simulink model "Microgrid_w_BESS"  (R2024b)
settings: Solver=VariableStepAuto  StartTime=0.0  StopTime=4  RelTol=1e-3
undefined symbols (not defined in the file or in its folder): Ion, Lithium, Ts_Control
libraries: spsParallelRLCBranchLib x8, simulink x6, spsSeriesRLCBranchLib x6, powerlib_extras x6, ee_lib x5, nesl_utility x5, slpidlib x5, spsThreePhaseVIMeasurementLib x3, spsThreePhaseSeriesRLCBranchLib x3, spsCurrentVoltageSimscapeInterfaceLib x3, eePowerMeasurement x3, spsVoltageMeasurementLib x2
(part 1 of 2)
settings Model: Creator=DELL  LastModifiedBy=mitphanase
settings DataIOCC: ReturnWorkspaceOutputs=off

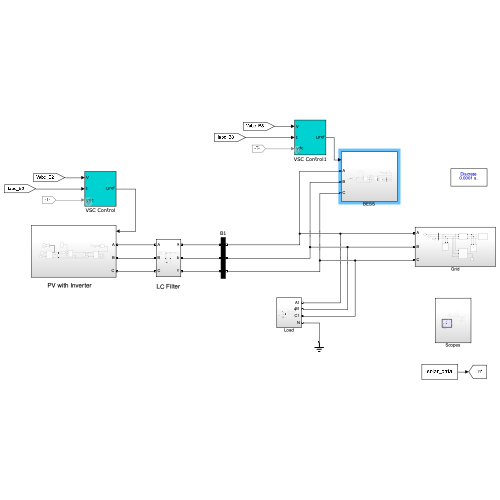
[thumbnail: Simulink's stored preview of the top-level diagram]
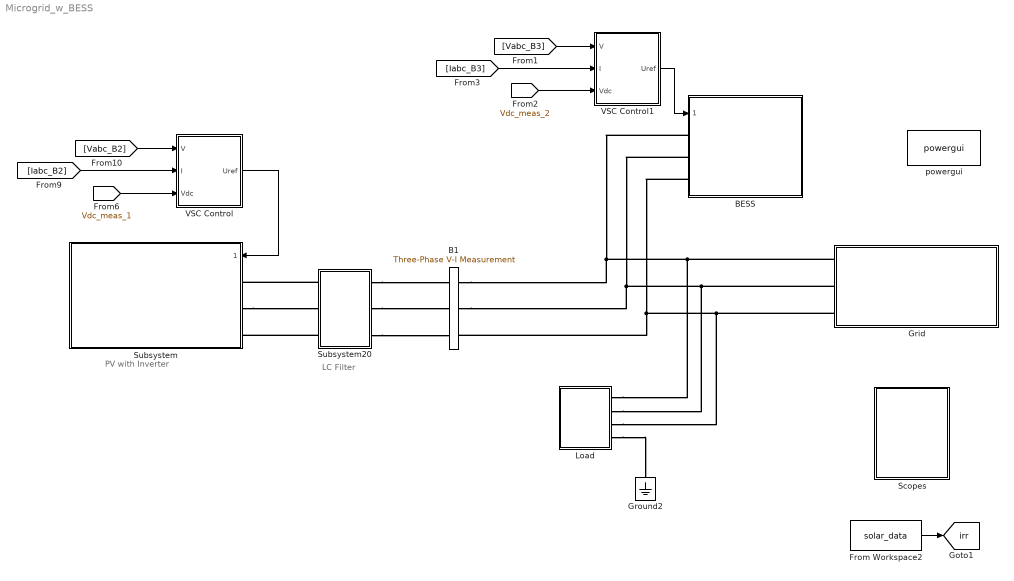
== system Microgrid_w_BESS ==
  note: LC Filter
  note: PV with Inverter
  B1 : spsThreePhaseVIMeasurementLib/Three-Phase V-I Measurement  VoltageMeasurement=phase-to-ground  SetLabelV=on  LabelV=Vabc_B1  Vpu=off  VpuLL=off  CurrentMeasurement=yes  SetLabelI=on  LabelI=Iabc_B1  Ipu=off  Pbase=100e6  Vbase=1000  OutputType=Magnitude  PhasorSimulation=off  PSBequivalent=0
  BESS : Subsystem
  From Workspace2 : FromWorkspace  VariableName=solar_data  OutDataTypeStr=double  SampleTime=0.01
  Grid : Subsystem
  Ground2 : spsGroundLib/Ground  LConnTagsString=a
  Load : Subsystem
  Scopes : Subsystem
  Subsystem : Subsystem
  Subsystem20 : Subsystem
  VSC Control : Subsystem  mask(VSC Main Controller){nom=[ 50e3  50 ], Vnom=[ 400 400 ], Vnom_dc=700, RLxfo=[0  0 ], RLchoke=[0  0  ], K_VDCreg=[18  600], K_Ireg=[0.2 20], Ts=Ts_Control}
      mask prompts: nom "Nominal power and frequency [ Pnom(VA)  Fnom(Hz) ]:"; Vnom "Nominal primary and secondary voltages (Vrms LL) [ Vnom_prim   Vnom_sec ]:"; Vnom_dc "Nominal DC bus voltage (V):"; RLxfo "Total transformer leakage impedance (pu/Pnom) [ Rxfo  Lxf ]"; RLchoke "Choke impedance [ R(ohm) L(H) ]"; K_VDCreg "VDC regultator gains [ Kp  Ki ]:"; K_Ireg "Current regulator gains [ Kp  Ki ]:"; Ts "Sample time"
      mask init:
      | Pnom=nom(1);
      | Fnom=nom(2);
      | Vnom_prim=Vnom(1);
      | Vnom_sec=Vnom(2);
      | Zbase=Vnom_sec^2/Pnom;
      | Rtot_pu=RLxfo(1) + RLchoke(1)/Zbase;
      | Ltot_pu=RLxfo(2) + RLchoke(2)/(Zbase/(2*pi*Fnom));
      | Kp_VDCreg=K_VDCreg(1);
      | Ki_VDCreg=K_VDCreg(2);
      | Kp_Ireg=K_Ireg(1);
      | Ki_Ireg=K_Ireg(2);
      | Vdc_ref=Vnom_dc;
  VSC Control1 : Subsystem  mask(VSC Main Controller){nom=[ 45e3  50 ], Vnom=[ 400 400 ], Vnom_dc=600, RLxfo=[0  0 ], RLchoke=[0  0  ], K_VDCreg=[18  600], K_Ireg=[0.2 20], Ts=Ts_Control}
      mask prompts: nom "Nominal power and frequency [ Pnom(VA)  Fnom(Hz) ]:"; Vnom "Nominal primary and secondary voltages (Vrms LL) [ Vnom_prim   Vnom_sec ]:"; Vnom_dc "Nominal DC bus voltage (V):"; RLxfo "Total transformer leakage impedance (pu/Pnom) [ Rxfo  Lxf ]"; RLchoke "Choke impedance [ R(ohm) L(H) ]"; K_VDCreg "VDC regultator gains [ Kp  Ki ]:"; K_Ireg "Current regulator gains [ Kp  Ki ]:"; Ts "Sample time"
      mask init: same as Microgrid_w_BESS/VSC Control
  powergui : sps_lib/powergui  Priority=1  SimulationMode=Discrete  SampleTime=1e-4  frequency=60  Iterations=50  frequencyindice=0  Pbase=100e6  ErrMax=1e-4  UnitsV=kV  UnitsW=MW  buscounter=0  FunctionMessages=off  echomessages=off  EnableUseOfTLC=off  CurrentSourceSwitches=off  DisableSnubberDevices=off  DisableRonSwitches=off  DisableVfSwitches=off  DisplayEquations=off  AutomaticDiscreteSolvers=off  SolverType=Tustin/Backward Euler (TBE)  Interpol=off  ExternalGateDelay=off  methode=off  Ts=100  x0status=blocks  SPID=on  SwTol=0  HookPort=off  NonlinearTolerance=1e-4  nMaxIteration=100  ContinueOnMaxIteration=off  RestoreLinks=warning  ResistiveCurrentMeasurement=off  Frange=[0:2:500]  Ylog=off  Xlog=on  ShowGrid=off  save=off  variable=ZData  structure=0  ZoomFFT=off  StartTime=0.0  cycles=1  DisplayStyle=1  fundamental=60  FreqAxis=off  MaxFrequency=1000  frequencyindicesteady=1  RmsSteady=1  display=off
  tag scope: irr=global
  wires:
  [Vdc_meas_1] -> VSC Control/3(Vdc)
  [Vabc_B2] -> VSC Control/1(V)
  [Iabc_B2] -> VSC Control/2(I)
  VSC Control/1(Uref) -> Subsystem/1("  ")
  From Workspace2/1 -> [irr]
  [Iabc_B3] -> VSC Control1/2(I)
  [Vabc_B3] -> VSC Control1/1(V)
  [Vdc_meas_2] -> VSC Control1/3(Vdc)
  VSC Control1/1(Uref) -> BESS/1("  ")
  connections:
  Grid/LConn1 -- Load/LConn1 -- B1/RConn1 -- BESS/LConn1
  Grid/LConn3 -- Load/LConn3 -- BESS/LConn3 -- B1/RConn3
  Grid/LConn2 -- Load/LConn2 -- B1/RConn2 -- BESS/LConn2
  Subsystem20/LConn1 -- Subsystem/LConn1
  Subsystem/LConn2 -- Subsystem20/LConn2
  Subsystem20/LConn3 -- Subsystem/LConn3
  Subsystem20/RConn1 -- B1/LConn1
  Subsystem20/RConn2 -- B1/LConn2
  Subsystem20/RConn3 -- B1/LConn3
  Load/LConn4 -- Ground2/LConn1

== system Microgrid_w_BESS/BESS ==
  "  " : Inport
  B3 : spsThreePhaseVIMeasurementLib/Three-Phase V-I Measurement  VoltageMeasurement=phase-to-ground  SetLabelV=on  LabelV=Vabc_B3  Vpu=off  VpuLL=off  CurrentMeasurement=yes  SetLabelI=on  LabelI=Iabc_B3  Ipu=off  Pbase=100e6  Vbase=1000  OutputType=Magnitude  PhasorSimulation=off  PSBequivalent=0
  BATT chg-dshg logic1 : Subsystem
  Battery : spsBatteryLib/Battery  BatType=Lithium-Ion  NomV=400  NomQ=150  SOC=0  Batt_Tr=0.01  PresetModel=on  MaxQ=150  MinV=300  FullV=465.5949  Dis_rate=65.2174  R=0.026667  Normal_OP=135.6522  expZone="[432.1543      7.369565]"
  Current Measurement : spsCurrentMeasurementLib/Current Measurement  PhasorSimulation=off  OutputType=Complex  PSBequivalent=0
  Inverter ON/OFF Logic : Subsystem
  L_B : spsSeriesRLCBranchLib/Series RLC Branch  LConnTagsString=__new0  RConnTagsString=__new0  BranchType=L  Resistance=5e-3  Inductance=1e-3  SetiL0=off  InitialCurrent=0  Capacitance=100e-6  Setx0=off  InitialVoltage=230  Measurements=None
  Subsystem : Subsystem
  Subsystem20 : Subsystem
  Two-Level Converter : spsTwoLevelConverterLib/Two-Level Converter  ModelType=Average model (No rectifier mode)  Ron=1e-3  Rs=1e6  Cs=inf  Vforward=[0,0]  Ron_Diode=1e-3  Rs_Diode=1e6  Cs_Diode=inf  Vf_Diode=1e-3  Rs_CurrentSource=inf  Ron_ACsource=1e-3
      settings: LibrarySourceBlock=sps_lib/Power Electronics/Two-Level Converter
  Two-Quadrant DC/DC Converter : spsTwoQuadrantDCDCConverterLib/Two-Quadrant DC//DC Converter  ModelType=Average model (D-controlled)  Ron=1e-3  Rs=1e6  Cs=inf  Vforward=[0,0]  Ron_Diode=1e-3  Rs_Diode=1e6  Cs_Diode=inf  Vf_Diode=1e-3  Rs_CurrentSource=inf  Ron_ACsource=1e-3
  A : PMIOPort  Side=Left
  B : PMIOPort  Port=2  Side=Left
  C : PMIOPort  Port=3  Side=Left
  tag scope: Batt_m=global
  wires:
  BATT chg-dshg logic1/1(D) -> Two-Quadrant DC/DC Converter/1
  [Vdc_meas_2] -> Inverter ON/OFF Logic/1(V_DC)
  "  "/1 -> Inverter ON/OFF Logic/2(g_in)
  Inverter ON/OFF Logic/1(g_out) -> Two-Level Converter/1
  Battery/1 -> [Batt_m]
  connections:
  Two-Level Converter/RConn2 -- Subsystem/RConn2 -- Two-Quadrant DC/DC Converter/RConn2 -- Battery/LConn2
  L_B/RConn1 -- Two-Quadrant DC/DC Converter/LConn1
  Subsystem/RConn1 -- Two-Level Converter/RConn1 -- Two-Quadrant DC/DC Converter/RConn1
  Subsystem20/LConn2 -- Two-Level Converter/LConn2
  Two-Level Converter/LConn1 -- Subsystem20/LConn1
  Two-Level Converter/LConn3 -- Subsystem20/LConn3
  Current Measurement/RConn1 -- Battery/LConn1
  Current Measurement/LConn1 -- L_B/LConn1
  B3/LConn1 -- Subsystem20/RConn1
  B3/LConn2 -- Subsystem20/RConn2
  B3/LConn3 -- Subsystem20/RConn3
  B3/RConn1 -- A/RConn1
  B3/RConn2 -- B/RConn1
  B3/RConn3 -- C/RConn1

== system Microgrid_w_BESS/Grid ==
  B2 : spsThreePhaseVIMeasurementLib/Three-Phase V-I Measurement  VoltageMeasurement=phase-to-ground  SetLabelV=on  LabelV=Vabc_B2  Vpu=off  VpuLL=off  CurrentMeasurement=yes  SetLabelI=on  LabelI=Iabc_B2  Ipu=off  Pbase=100e6  Vbase=500e3  OutputType=Magnitude  PhasorSimulation=off  PSBequivalent=0
  Ground : spsGroundLib/Ground  LConnTagsString=a
  "Grounding Transformer " : spsGroundingTransformerLib/Grounding Transformer   UNITS=SI  NominalPower="[3e3   50]"  NominalVoltage=0.4e3  ZeroSequenceImpedance_pu=[0.025 0.75]  MagnetizationBranch_pu=[500 500]  ZeroSequenceImpedance_SI=[1.3333 40]  MagnetizationBranch_SI=[26667 26667]  Measurements=All voltages and currents
      settings: LibrarySourceBlock=|
      | sps_lib/Power Grid Elements/Grounding
      | Transformer
  Three-Phase Series RLC Branch3 : spsThreePhaseSeriesRLCBranchLib/Three-Phase Series RLC Branch  LConnTagsString=A|B|C  RConnTagsString=A|B|C  BranchType=RL  Resistance=0.02  Inductance=1e-3  Capacitance=1e-6  Measurements=None
  Three-Phase Series RLC Load : spsThreePhaseSeriesRLCLoadLib/Three-Phase Series RLC Load  LConnTagsString=A|B|C  Configuration=Y (grounded)  NominalVoltage=400  Vabc=[1e3 1e3 1e3]  Vabcp=[1e3 1e3 1e3]  NominalFrequency=50  UnbalancedPower=off  ActivePower=0.1  InductivePower=0  CapacitivePower=100  Pabc=[10e3 9e3 11e3]  QLabc=[100 90 110]  QCabc=[100 90 110]  Pabcp=[10e3 9e3 11e3]  QLabcp=[100 90 110]  QCabcp=[100 90 110]  Measurements=None  LoadType=constant Z
  Three-Phase Series RLC Load1 : spsThreePhaseSeriesRLCLoadLib/Three-Phase Series RLC Load  LConnTagsString=A|B|C  Configuration=Y (grounded)  NominalVoltage=400  Vabc=[1e3 1e3 1e3]  Vabcp=[1e3 1e3 1e3]  NominalFrequency=50  UnbalancedPower=off  ActivePower=10  InductivePower=0  CapacitivePower=0  Pabc=[10e3 9e3 11e3]  QLabc=[100 90 110]  QCabc=[100 90 110]  Pabcp=[10e3 9e3 11e3]  QLabcp=[100 90 110]  QCabcp=[100 90 110]  Measurements=None  LoadType=constant Z
  Three-Phase Source : spsThreePhaseSourceLib/Three-Phase Source  InternalConnection=Yg  VoltagePhases=off  Voltage=400  PhaseAngle=0  Voltage_phases=[25e3 25e3 25e3]/sqrt(3)  PhaseAngles_phases=[0 -120 +120]  Frequency=50  NonIdealSource=on  SpecifyImpedance=on  Resistance=0.0113  Inductance=36e-6  ShortCircuitLevel=10e6  BaseVoltage=400  XRratio=6  BusType=swing  Pref=10e3  Qref=0  Prefabc=[10e3, 10e3, 10e3]  Qrefabc=[0, 0, 0]  Qmin=-inf  Qmax=inf
  A : PMIOPort  Side=Left
  B : PMIOPort  Port=2  Side=Left
  C : PMIOPort  Port=3  Side=Left
  connections:
  "Grounding Transformer "/RConn1 -- Ground/LConn1
  Three-Phase Series RLC Load/LConn1 -- Three-Phase Series RLC Branch3/RConn1 -- Three-Phase Source/RConn1
  Three-Phase Series RLC Load/LConn2 -- Three-Phase Series RLC Branch3/RConn2 -- Three-Phase Source/RConn2
  Three-Phase Series RLC Load/LConn3 -- Three-Phase Series RLC Branch3/RConn3 -- Three-Phase Source/RConn3
  "Grounding Transformer "/LConn1 -- B2/LConn1 -- Three-Phase Series RLC Load1/LConn1 -- Three-Phase Series RLC Branch3/LConn1
  "Grounding Transformer "/LConn2 -- Three-Phase Series RLC Load1/LConn2 -- B2/LConn2 -- Three-Phase Series RLC Branch3/LConn2
  "Grounding Transformer "/LConn3 -- Three-Phase Series RLC Load1/LConn3 -- B2/LConn3 -- Three-Phase Series RLC Branch3/LConn3
  B2/RConn3 -- C/RConn1
  B2/RConn2 -- B/RConn1
  B2/RConn1 -- A/RConn1

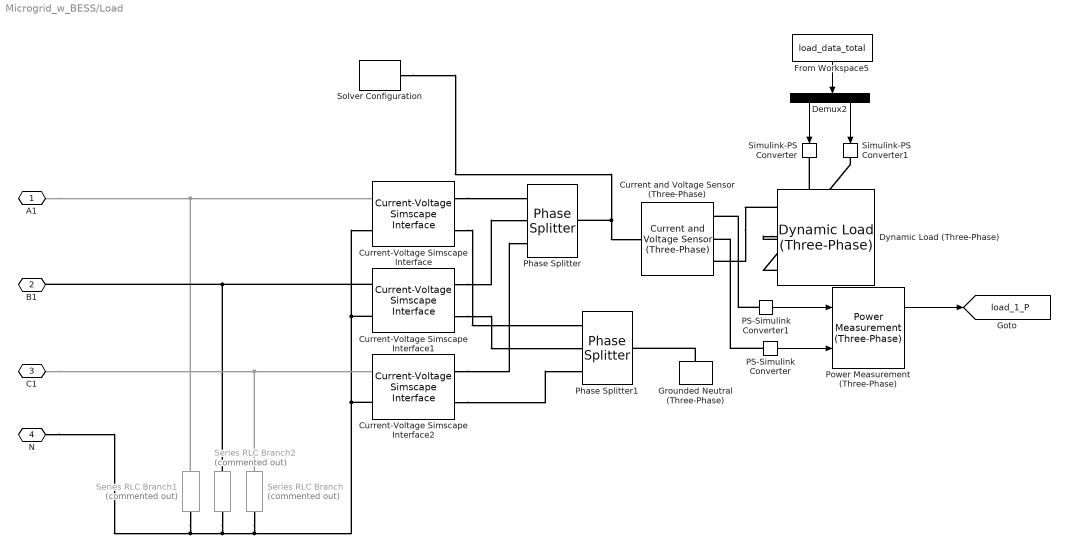
== system Microgrid_w_BESS/Load ==
  Current and Voltage Sensor (Three-Phase) : ee_lib/Sensors & Transducers/Current and Voltage Sensor (Three-Phase)  vMeasurementType=ee.enum.vmeasurement.ll  outputUnit=ee.enum.unit.si  SRated=100e6 A*V  VRated=24e3 V  I_specify=off  I_priority=None  I=[0, 0, 0] A  I_nominal_specify=off  I_nominal_value=1  I_nominal_unit=A  V_specify=off  V_priority=None  V=[0, 0, 0] V  V_nominal_specify=off  V_nominal_value=1  V_nominal_unit=V
      settings: InternalSimscapePortConfiguration="{\"Bottom\":[],\"Left\":[{\"id\":\"N1\",\"label\":\"~1\",\"type\":\"foundation.electrical.three_phase\"}],\"Right\":[{\"id\":\"V_output\",\"label\":\"V\",\"type\":\"output\"},{\"id\":\"I_output\",\"label\":\"I\",\"type\":\"output\"},{\"id\":\"N2\",\"label\":\"~2\",\"type\":\"foundation.electrical.three_phase\"}],\"Top\":[]}"
  Current-Voltage Simscape Interface : spsCurrentVoltageSimscapeInterfaceLib/Current-Voltage Simscape Interface  DFT=off  FMode=Low pass filter (continuous)  T=1e-4  Ts=50e-6  i0=0  v0=0  Sd=Specialized Power Systems side  Measurements=off
  Current-Voltage Simscape Interface1 : spsCurrentVoltageSimscapeInterfaceLib/Current-Voltage Simscape Interface  DFT=off  FMode=Low pass filter (continuous)  T=1e-4  Ts=50e-6  i0=0  v0=0  Sd=Specialized Power Systems side  Measurements=off
  Current-Voltage Simscape Interface2 : spsCurrentVoltageSimscapeInterfaceLib/Current-Voltage Simscape Interface  DFT=off  FMode=Low pass filter (continuous)  T=1e-4  Ts=50e-6  i0=0  v0=0  Sd=Specialized Power Systems side  Measurements=off
  Demux2 : Demux  Outputs=2
  Dynamic Load (Three-Phase) : ee_lib/Passive/Dynamic Load (Three-Phase)  port_option=ee.enum.threePhasePort.composite  FRated=50 Hz  Vline_rms_min=1 V  tau=0.01 s  Vline_rms_ini=400 V  Vang_ini=0 deg  gmin=0 S  fault_action=simscape.enum.assert.action.none  t_fault=1 s
      settings: InternalSimscapePortConfiguration="{\"Bottom\":[],\"Left\":[{\"id\":\"N\",\"label\":\"~\",\"type\":\"foundation.electrical.three_phase\"}],\"Right\":[],\"Top\":[{\"id\":\"P\",\"label\":\"P\",\"type\":\"input\"},{\"id\":\"Q\",\"label\":\"Q\",\"type\":\"input\"}]}"
  From Workspace5 : FromWorkspace  VariableName=load_data_total  SampleTime=0.01
  Grounded Neutral (Three-Phase) : ee_lib/Connectors & References/Grounded Neutral (Three-Phase)
  PS-Simulink Converter : nesl_utility/PS-Simulink Converter  PhysicalDomain=network_engine_domain  SubClassName=ps_output  LeftPortType=input  RightPortType=output  PseudoPeriodic=off  Frequencies=[]  VectorFormat=inherit  Unit=inherit  AffineConversion=off
  PS-Simulink Converter1 : nesl_utility/PS-Simulink Converter  PhysicalDomain=network_engine_domain  SubClassName=ps_output  LeftPortType=input  RightPortType=output  PseudoPeriodic=off  Frequencies=[]  VectorFormat=inherit  Unit=inherit  AffineConversion=off
  Phase Splitter : ee_lib/Connectors & References/Phase Splitter
  Phase Splitter1 : ee_lib/Connectors & References/Phase Splitter
  Power Measurement (Three-Phase) : eePowerMeasurement/Power Measurement (Three-Phase)  LabelModeActiveChoice=Discrete  F=50  K=[1]  Seq=Positive  Ts=0.01
  Series RLC Branch : spsSeriesRLCBranchLib/Series RLC Branch  Commented=on  LConnTagsString=__new0  RConnTagsString=__new0  BranchType=R  Resistance=1  Inductance=1e-3  SetiL0=off  InitialCurrent=0  Capacitance=1e-6  Setx0=off  InitialVoltage=0  Measurements=None
  Series RLC Branch1 : spsSeriesRLCBranchLib/Series RLC Branch  Commented=on  LConnTagsString=__new0  RConnTagsString=__new0  BranchType=R  Resistance=1  Inductance=1e-3  SetiL0=off  InitialCurrent=0  Capacitance=1e-6  Setx0=off  InitialVoltage=0  Measurements=None
  Series RLC Branch2 : spsSeriesRLCBranchLib/Series RLC Branch  Commented=on  LConnTagsString=__new0  RConnTagsString=__new0  BranchType=R  Resistance=1  Inductance=1e-3  SetiL0=off  InitialCurrent=0  Capacitance=1e-6  Setx0=off  InitialVoltage=0  Measurements=None
  Simulink-PS Converter : nesl_utility/Simulink-PS Converter  PhysicalDomain=network_engine_domain  SubClassName=ps_input  LeftPortType=input  RightPortType=output  PseudoPeriodic=off  Frequencies=[]  NoiseDistribution=none  NoiseParameters=[]  Unit=1  AffineConversion=off  FilteringAndDerivatives=provide  SimscapeFilterOrder=1  InputFilterTimeConstant=0.001  UdotUserProvided=0
  Simulink-PS Converter1 : nesl_utility/Simulink-PS Converter  PhysicalDomain=network_engine_domain  SubClassName=ps_input  LeftPortType=input  RightPortType=output  PseudoPeriodic=off  Frequencies=[]  NoiseDistribution=none  NoiseParameters=[]  Unit=1  AffineConversion=off  FilteringAndDerivatives=provide  SimscapeFilterOrder=1  InputFilterTimeConstant=0.001  UdotUserProvided=0
  Solver Configuration : nesl_utility/Solver Configuration  PhysicalDomain=network_engine_domain  SubClassName=solver  LeftPortType=input  RightPortType=generic  Tones=[]  Harmonics=[]  SimulateNoise=off  Profile=off  UseLocalSampling=off  EnableSwitchedLinearOptims=on  FrequencyDomain=off  UseCCode=off  RelTol=0.001  AbsTol=0.001  MinStep=1e-09  ToWorkspace=off  RevertToSquareIcSolve=off  NumHomotopyIterations=100  PhasorMode=off  PhasorModeNumHarmonics=1  ConsistencySolver=NEWTON_XTOL_AFTER_FTOL  IndexReductionMethod=DerivativeReplacement  DoDC=on  ResidualTolerance=1e-09  ConsistencyTolSource=GLOBAL  ConsistencyAbsTol=0.001  ConsistencyRelTol=0.001  ConsistencyTolFactor=0.001  UseLocalSolver=off  LocalSolverChoice=NE_BACKWARD_EULER_ADVANCER  ResolveIndetEquations=on  FunctionEvalNumThread=1  LocalSolverSampleTime=0.0001  DoFixedCost=off  MaxNonlinIter=3  MaxModeIter=2  ComputeImpulses=off  ImpulseIterations=2  LinearAlgebra=Sparse  LinearAlgebraNumThread=0  EquationFormulation=NE_TIME_EF  DelaysMemoryBudget=1024  AutomaticFiltering=off  FilteringTimeConstant=0.001  PartitionStorageMethod=AS_NEEDED  PartitionMemoryBudget=1024  PartitionMethod=ROBUST  MultibodyUseLocalSolver=off  MultibodyLocalSolverChoice=ODE1  MultibodyLocalSolverSampleTime=0.001
  A1 : PMIOPort  Side=Left
  B1 : PMIOPort  Port=2  Side=Left
  C1 : PMIOPort  Port=3  Side=Left
  N : PMIOPort  Port=4  Side=Left
  tag scope: load_1_P=global
  wires:
  From Workspace5/1 -> Demux2/1
  Demux2/2 -> Simulink-PS Converter1/1
  Demux2/1 -> Simulink-PS Converter/1
  PS-Simulink Converter1/1 -> Power Measurement (Three-Phase)/1
  PS-Simulink Converter/1 -> Power Measurement (Three-Phase)/2
  Power Measurement (Three-Phase)/1 -> [load_1_P]
  connections:
  Solver Configuration/RConn1 -- Current and Voltage Sensor (Three-Phase)/LConn1 -- Phase Splitter/LConn1
  Current-Voltage Simscape Interface1/RConn2 -- Phase Splitter1/RConn2
  Current-Voltage Simscape Interface2/RConn2 -- Phase Splitter1/RConn3
  Dynamic Load (Three-Phase)/LConn1 -- Current and Voltage Sensor (Three-Phase)/RConn3
  Current-Voltage Simscape Interface1/RConn1 -- Phase Splitter/RConn2
  Current-Voltage Simscape Interface2/RConn1 -- Phase Splitter/RConn3
  Current-Voltage Simscape Interface/RConn1 -- Phase Splitter/RConn1
  Dynamic Load (Three-Phase)/LConn3 -- Simulink-PS Converter1/RConn1
  Grounded Neutral (Three-Phase)/LConn1 -- Phase Splitter1/LConn1
  Current-Voltage Simscape Interface/RConn2 -- Phase Splitter1/RConn1
  Dynamic Load (Three-Phase)/LConn2 -- Simulink-PS Converter/RConn1
  Series RLC Branch1/LConn1 -- Current-Voltage Simscape Interface/LConn1 -- A1/RConn1
  Current-Voltage Simscape Interface1/LConn1 -- Series RLC Branch2/LConn1 -- B1/RConn1
  Current-Voltage Simscape Interface1/LConn2 -- Series RLC Branch/RConn1 -- N/RConn1 -- Series RLC Branch1/RConn1 -- Series RLC Branch2/RConn1 -- Current-Voltage Simscape Interface2/LConn2 -- Current-Voltage Simscape Interface/LConn2
  Series RLC Branch/LConn1 -- C1/RConn1 -- Current-Voltage Simscape Interface2/LConn1
  PS-Simulink Converter1/LConn1 -- Current and Voltage Sensor (Three-Phase)/RConn1
  PS-Simulink Converter/LConn1 -- Current and Voltage Sensor (Three-Phase)/RConn2

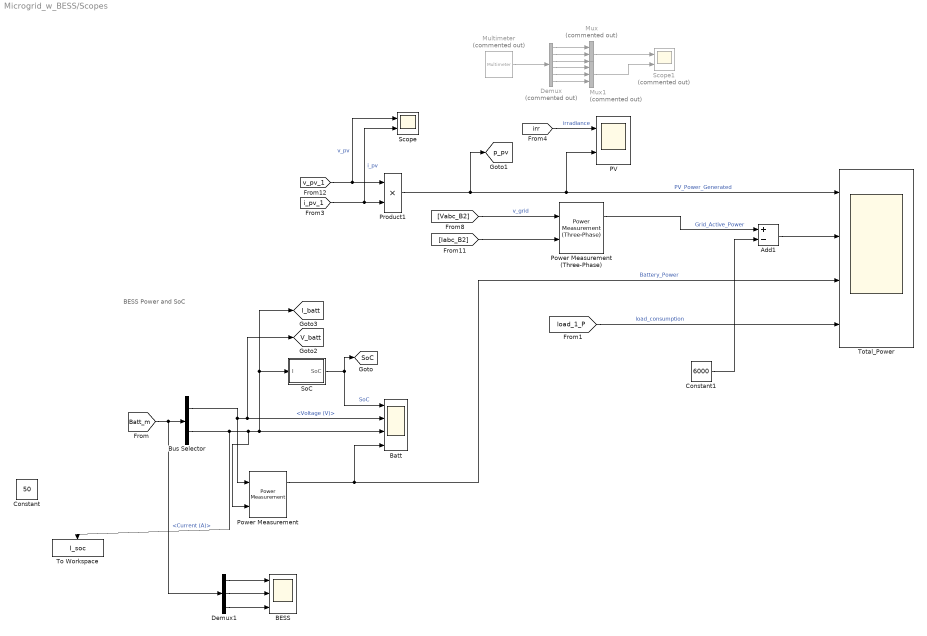
== system Microgrid_w_BESS/Scopes ==
  note: BESS Power and SoC
  Add1 : Sum  Inputs=+-
  BESS : Scope  NumInputPorts=3
  Batt : Scope  NumInputPorts=4
  Bus Selector : BusSelector  OutputSignals=Voltage (V),Current (A)
  Constant : Constant  Value=50
  Constant1 : Constant  Value=6000
  Demux : Demux  Commented=on  Outputs=6
  Demux1 : Demux  Outputs=3
  Multimeter : spsMultimeterLib/Multimeter  Commented=on  L=2  sel=1  yselected={}  Gain=0  OutputType=Complex  PlotAtSimulationStop=off  PhasorSimulation=off
  Mux : Mux  Commented=on  Inputs=3
  Mux1 : Mux  Commented=on  Inputs=3
  PV : Scope  NumInputPorts=2
  Power Measurement : eePowerMeasurement/Power Measurement  LabelModeActiveChoice=Discrete  F=50  K=[0]  Ts=0.001
  Power Measurement (Three-Phase) : eePowerMeasurement/Power Measurement (Three-Phase)  LabelModeActiveChoice=Discrete  F=50  K=[1]  Seq=Positive  Ts=Ts_Control
  Product1 : Product
  Scope : Scope  NumInputPorts=2
  Scope1 : Scope  Commented=on  NumInputPorts=2
  SoC : Subsystem
  To Workspace : ToWorkspace  VariableName=I_soc  SaveFormat=Timeseries  SampleTime=0.01
  Total_Power : Scope  NumInputPorts=4
  tag scope: I_batt=global, SoC=global, V_batt=global, p_pv=global
  wires:
  [irr] -> PV/1  "irradiance"
  SoC/1(SoC) -> [SoC], Batt/1  "SoC"
  [Batt_m] -> Bus Selector/1, Demux1/1
  Power Measurement/1 -> Total_Power/3, Batt/4  "Battery_Power"
  [Vabc_B2] -> Power Measurement (Three-Phase)/1  "v_grid"
  [Iabc_B2] -> Power Measurement (Three-Phase)/2
  [load_1_P] -> Total_Power/4  "load_consumption"
  Multimeter/1 -> Demux/1
  Demux/1 -> Mux/1
  Demux/2 -> Mux/2
  Mux/1 -> Scope1/1
  Demux/3 -> Mux/3
  Demux/4 -> Mux1/1
  Demux/5 -> Mux1/2
  Demux/6 -> Mux1/3
  Mux1/1 -> Scope1/2
  [i_pv_1] -> Scope/2, Product1/2  "i_pv"
  [v_pv_1] -> Scope/1, Product1/1  "v_pv"
  Product1/1 -> [p_pv], PV/2, Total_Power/1  "PV_Power_Generated"
  Bus Selector/1 -> [V_batt], Batt/2, Power Measurement/1  "<Voltage (V)>"
  Power Measurement (Three-Phase)/1 -> Add1/1  "Grid_Active_Power"
  Add1/1 -> Total_Power/2
  Constant1/1 -> Add1/2
  Demux1/1 -> BESS/1
  Demux1/2 -> BESS/2
  Demux1/3 -> BESS/3
  Bus Selector/2 -> Power Measurement/2, Batt/3, SoC/1(I), [I_batt], To Workspace/1  "<Current (A)>"

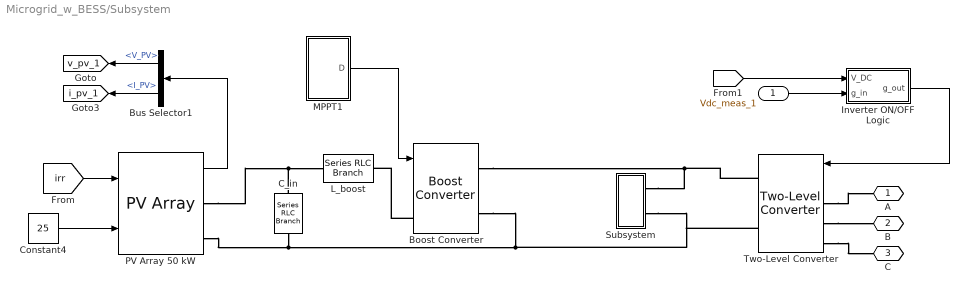
== system Microgrid_w_BESS/Subsystem ==
  "  " : Inport
  Boost Converter : spsBoostConverterLib/Boost Converter  ModelType=Average model (D-controlled)  Ron=1e-3  Rs=1e6  Cs=inf  Vforward=[0,0]  Ron_Diode=1e-3  Rs_Diode=1e6  Cs_Diode=inf  Vf_Diode=1e-3  Rs_CurrentSource=inf  Ron_ACsource=1e-3
      settings: LibrarySourceBlock=sps_lib/Power Electronics/Boost Converter
  Bus Selector1 : BusSelector  OutputSignals=V_PV,I_PV
  C_in : spsSeriesRLCBranchLib/Series RLC Branch  LConnTagsString=__new0  RConnTagsString=__new0  BranchType=C  Resistance=1e-5  Inductance=1e-3  SetiL0=off  InitialCurrent=0  Capacitance=2515e-6  Setx0=off  InitialVoltage=426.5  Measurements=Branch voltage and current
  Constant4 : Constant  Value=25
  Inverter ON/OFF Logic : Subsystem
  L_boost : spsSeriesRLCBranchLib/Series RLC Branch  LConnTagsString=__new0  RConnTagsString=__new0  BranchType=L  Resistance=1e-3  Inductance=20e-3  SetiL0=off  InitialCurrent=0  Capacitance=100e-6  Setx0=off  InitialVoltage=230  Measurements=None
  MPPT1 : Subsystem
  PV Array 50 kW : spsPVArrayLib/PV Array  Npar=24  Nser=5  PlotType=array @ 1000 W/m2 & specified temperatures  S_vec="[ 1000  500  100 ]"  Temp_C_vec="[ 45 25  ]"  ModuleName=SunPower SPR-415E-WHT-D  PlotWhenSelected=off  Pm=414.801  Ncell=128  Voc=85.3  Isc=6.09  Vm=72.9  Im=5.69  beta_Voc_pc=-0.229  alpha_Isc_pc=0.030706  beta_Voc=-0.19534  alpha_Isc=0.00187  IL=6.0978  I0=7.1698e-13  nI=0.87223  Rsh=419.7781  Rs=0.53711  RobustModel=off  RobustCellTemperature=313.3991  BAL=on  Tc=1e-6  Tfilter=5e-5
  Subsystem : Subsystem
  Two-Level Converter : spsTwoLevelConverterLib/Two-Level Converter  ModelType=Average model (No rectifier mode)  Ron=1e-3  Rs=1e6  Cs=inf  Vforward=[0,0]  Ron_Diode=1e-3  Rs_Diode=1e6  Cs_Diode=inf  Vf_Diode=1e-3  Rs_CurrentSource=inf  Ron_ACsource=1e-3
      settings: LibrarySourceBlock=sps_lib/Power Electronics/Two-Level Converter
  A : PMIOPort  Side=Left
  B : PMIOPort  Port=2  Side=Left
  C : PMIOPort  Port=3  Side=Left
  tag scope: i_pv_1=global, v_pv_1=global
  wires:
  Bus Selector1/1 -> [v_pv_1]  "<V_PV>"
  Bus Selector1/2 -> [i_pv_1]  "<I_PV>"
  PV Array 50 kW/1 -> Bus Selector1/1
  [irr] -> PV Array 50 kW/1
  MPPT1/1(D) -> Boost Converter/1
  "  "/1 -> Inverter ON/OFF Logic/2(g_in)
  Inverter ON/OFF Logic/1(g_out) -> Two-Level Converter/1
  Constant4/1 -> PV Array 50 kW/2
  [Vdc_meas_1] -> Inverter ON/OFF Logic/1(V_DC)
  connections:
  Two-Level Converter/LConn1 -- A/RConn1
  PV Array 50 kW/RConn2 -- C_in/RConn1 -- Two-Level Converter/RConn2 -- Subsystem/RConn2 -- Boost Converter/RConn2
  PV Array 50 kW/RConn1 -- C_in/LConn1 -- L_boost/LConn1
  Boost Converter/RConn1 -- Two-Level Converter/RConn1 -- Subsystem/RConn1
  Two-Level Converter/LConn3 -- C/RConn1
  Two-Level Converter/LConn2 -- B/RConn1
  Boost Converter/LConn1 -- L_boost/RConn1

== system Microgrid_w_BESS/Subsystem20 ==
  Parallel RLC Branch : spsParallelRLCBranchLib/Parallel RLC Branch  LConnTagsString=a  RConnTagsString=__new0  BranchType=RC  Resistance=16  Inductance=1e-3  SetiL0=off  InitialCurrent=0  Capacitance=25e-6  Setx0=off  InitialVoltage=0  Measurements=None
  Parallel RLC Branch1 : spsParallelRLCBranchLib/Parallel RLC Branch  LConnTagsString=a  RConnTagsString=__new0  BranchType=RC  Resistance=16  Inductance=1e-3  SetiL0=off  InitialCurrent=0  Capacitance=25e-6  Setx0=off  InitialVoltage=0  Measurements=None
  Parallel RLC Branch2 : spsParallelRLCBranchLib/Parallel RLC Branch  LConnTagsString=a  RConnTagsString=__new0  BranchType=RC  Resistance=16  Inductance=1e-3  SetiL0=off  InitialCurrent=0  Capacitance=25e-6  Setx0=off  InitialVoltage=0  Measurements=None
  Three-Phase Series RLC Branch1 : spsThreePhaseSeriesRLCBranchLib/Three-Phase Series RLC Branch  LConnTagsString=A|B|C  RConnTagsString=A|B|C  BranchType=L  Resistance=1  Inductance=3*0.13e-3  Capacitance=1e-6  Measurements=None
  A : PMIOPort  Side=Left
  B : PMIOPort  Port=2  Side=Left
  C : PMIOPort  Port=3  Side=Left
  a : PMIOPort  Port=4  Side=Right
  b : PMIOPort  Port=5  Side=Right
  c : PMIOPort  Port=6  Side=Right
  connections:
  Parallel RLC Branch2/RConn1 -- Parallel RLC Branch1/LConn1 -- c/RConn1 -- Three-Phase Series RLC Branch1/RConn3
  Three-Phase Series RLC Branch1/LConn3 -- C/RConn1
  Three-Phase Series RLC Branch1/LConn2 -- B/RConn1
  Three-Phase Series RLC Branch1/LConn1 -- A/RConn1
  a/RConn1 -- Three-Phase Series RLC Branch1/RConn1 -- Parallel RLC Branch1/RConn1 -- Parallel RLC Branch/LConn1
  b/RConn1 -- Three-Phase Series RLC Branch1/RConn2 -- Parallel RLC Branch2/LConn1 -- Parallel RLC Branch/RConn1

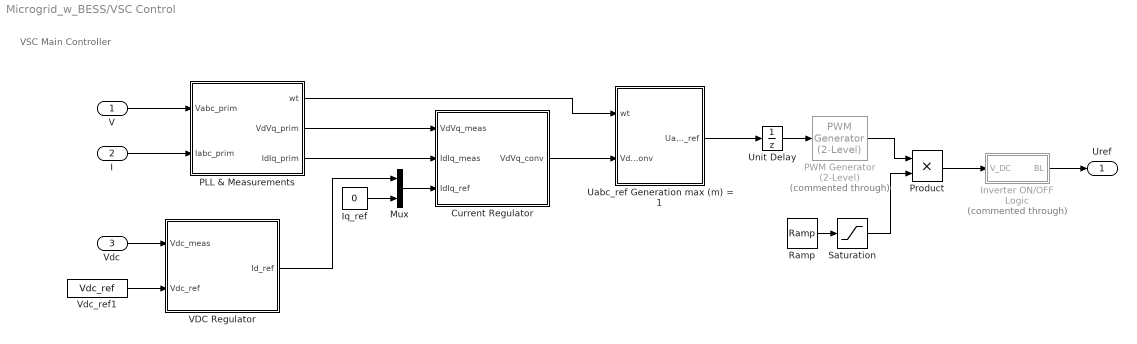
== system Microgrid_w_BESS/VSC Control ==
  note: VSC Main Controller
  V : Inport  PortDimensions=3
  I : Inport  Port=2  PortDimensions=3
  Vdc : Inport  Port=3  PortDimensions=1
  Current Regulator : Subsystem
  Inverter ON/OFF Logic : Subsystem  Commented=through
  Iq_ref : Constant  Value=0
  Mux : Mux  Inputs=2
  PLL & Measurements : Subsystem
  PWM Generator (2-Level) : spsPWMGenerator2LevelLib/PWM Generator (2-Level)  Commented=through  ModulatorType=Three-phase bridge (6 pulses)  ModulatorMode=Unsynchronized  Fc=27*50*8  Pc=90  nF=27  MinMax="[ -1  1 ]"  SamplingTechnique=Natural  ModulatingSignals=off  m=0.8  Freq=60  Phase=0  Ts=Ts_Control  ShowCarrierOutport=off
  Product : Product
  Ramp : simulink/Sources/Ramp  slope=1/0.02  start=0  InitialOutput=0
  Saturation : Saturate  UpperLimit=1  LowerLimit=0
  Uabc_ref Generation max (m) = 1 : Subsystem
  Unit Delay : UnitDelay  SampleTime=Ts_Control  HasFrameUpgradeWarning=on
  VDC Regulator : Subsystem
  Vdc_ref1 : Constant  Value=Vdc_ref
  Uref : Outport  VectorParamsAs1DForOutWhenUnconnected=off
  wires:
  Vdc_ref1/1 -> VDC Regulator/2(Vdc_ref)
  Uabc_ref Generation max (m) = 1/1(Uabc_ref) -> Unit Delay/1
  Unit Delay/1 -> PWM Generator (2-Level)/1
  I/1 -> PLL & Measurements/2(Iabc_prim)
  V/1 -> PLL & Measurements/1(Vabc_prim)
  Vdc/1 -> VDC Regulator/1(Vdc_meas)
  PLL & Measurements/2(VdVq_prim) -> Current Regulator/1(VdVq_meas)
  PLL & Measurements/3(IdIq_prim) -> Current Regulator/2(IdIq_meas)
  Mux/1 -> Current Regulator/3(IdIq_ref)
  Iq_ref/1 -> Mux/2
  PLL & Measurements/1(wt) -> Uabc_ref Generation max (m) = 1/1(wt)
  VDC Regulator/1(Id_ref) -> Mux/1
  PWM Generator (2-Level)/1 -> Product/1
  Current Regulator/1(VdVq_conv) -> Uabc_ref Generation max (m) = 1/2(VdVq_conv)
  Product/1 -> Inverter ON/OFF Logic/1(V_DC)
  Ramp/1 -> Saturation/1
  Saturation/1 -> Product/2
  Inverter ON/OFF Logic/1(BL) -> Uref/1

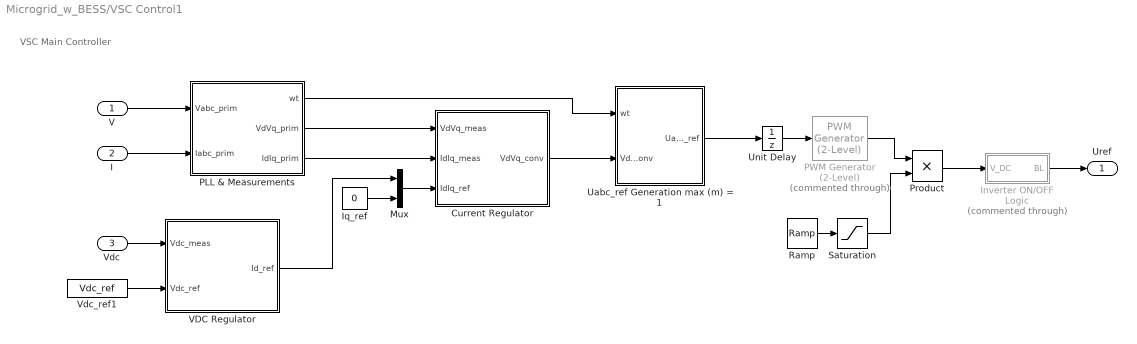
== system Microgrid_w_BESS/VSC Control1 ==
  note: VSC Main Controller
  V : Inport  PortDimensions=3
  I : Inport  Port=2  PortDimensions=3
  Vdc : Inport  Port=3  PortDimensions=1
  Current Regulator : Subsystem
  Inverter ON/OFF Logic : Subsystem  Commented=through
  Iq_ref : Constant  Value=0
  Mux : Mux  Inputs=2
  PLL & Measurements : Subsystem
  PWM Generator (2-Level) : spsPWMGenerator2LevelLib/PWM Generator (2-Level)  Commented=through  ModulatorType=Three-phase bridge (6 pulses)  ModulatorMode=Unsynchronized  Fc=27*50*8  Pc=90  nF=27  MinMax="[ -1  1 ]"  SamplingTechnique=Natural  ModulatingSignals=off  m=0.8  Freq=60  Phase=0  Ts=Ts_Control  ShowCarrierOutport=off
  Product : Product
  Ramp : simulink/Sources/Ramp  slope=1/0.02  start=0  InitialOutput=0
  Saturation : Saturate  UpperLimit=1  LowerLimit=0
  Uabc_ref Generation max (m) = 1 : Subsystem
  Unit Delay : UnitDelay  SampleTime=Ts_Control  HasFrameUpgradeWarning=on
  VDC Regulator : Subsystem
  Vdc_ref1 : Constant  Value=Vdc_ref
  Uref : Outport  VectorParamsAs1DForOutWhenUnconnected=off
  wires:
  Inverter ON/OFF Logic/1(BL) -> Uref/1
  Saturation/1 -> Product/2
  Ramp/1 -> Saturation/1
  Product/1 -> Inverter ON/OFF Logic/1(V_DC)
  Current Regulator/1(VdVq_conv) -> Uabc_ref Generation max (m) = 1/2(VdVq_conv)
  PWM Generator (2-Level)/1 -> Product/1
  VDC Regulator/1(Id_ref) -> Mux/1
  PLL & Measurements/1(wt) -> Uabc_ref Generation max (m) = 1/1(wt)
  Iq_ref/1 -> Mux/2
  Mux/1 -> Current Regulator/3(IdIq_ref)
  PLL & Measurements/3(IdIq_prim) -> Current Regulator/2(IdIq_meas)
  PLL & Measurements/2(VdVq_prim) -> Current Regulator/1(VdVq_meas)
  Vdc/1 -> VDC Regulator/1(Vdc_meas)
  V/1 -> PLL & Measurements/1(Vabc_prim)
  I/1 -> PLL & Measurements/2(Iabc_prim)
  Unit Delay/1 -> PWM Generator (2-Level)/1
  Uabc_ref Generation max (m) = 1/1(Uabc_ref) -> Unit Delay/1
  Vdc_ref1/1 -> VDC Regulator/2(Vdc_ref)

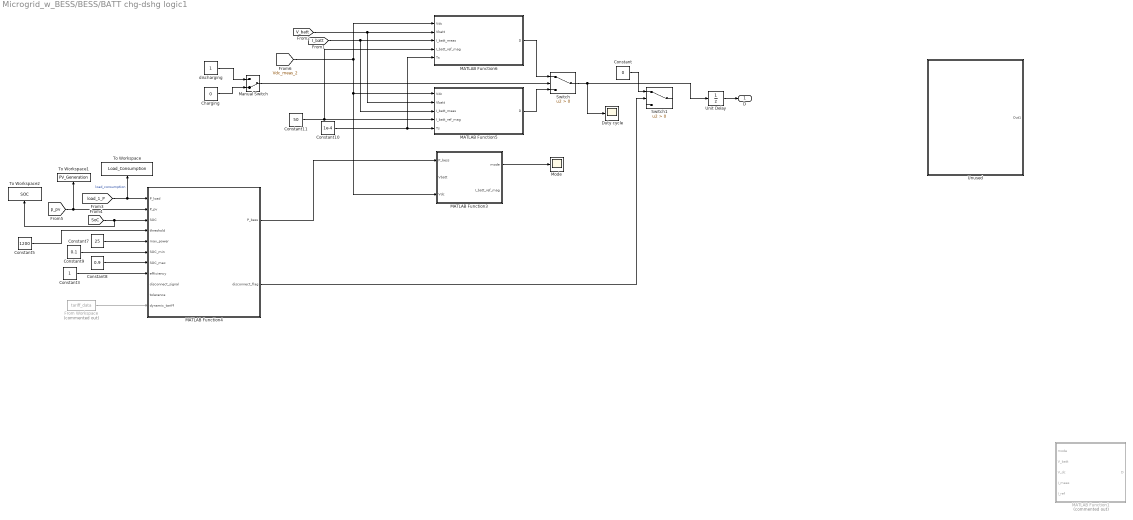
== system Microgrid_w_BESS/BESS/BATT chg-dshg logic1 ==
  Charging : Constant  Value=0
  Constant : Constant  Value=0
  Constant10 : Constant  Value=1e-4
  Constant11 : Constant  Value=50
  Constant3 : Constant
  Constant5 : Constant  Value=1200
  Constant7 : Constant  Value=25
  Constant8 : Constant  Value=0.9
  Constant9 : Constant  Value=0.1
  Duty cycle : Scope
  From Workspace : FromWorkspace  Commented=on  VariableName=tariff_data
  MATLAB Function1 : MATLAB Function  Commented=on  TreatAsAtomicUnit=on
  MATLAB Function3 : MATLAB Function  TreatAsAtomicUnit=on
  MATLAB Function4 : MATLAB Function  TreatAsAtomicUnit=on
  MATLAB Function5 : MATLAB Function  TreatAsAtomicUnit=on
  MATLAB Function6 : MATLAB Function  TreatAsAtomicUnit=on
  Manual Switch : ManualSwitch  CurrentSetting=0
  Mode : Scope
  Switch : Switch  Criteria=u2 > Threshold  SaturateOnIntegerOverflow=off  InputSameDT=off
  Switch1 : Switch  Criteria=u2 > Threshold  SaturateOnIntegerOverflow=off  InputSameDT=off
  To Workspace : ToWorkspace  VariableName=Load_Consumption  SaveFormat=Timeseries  SampleTime=-1
  To Workspace1 : ToWorkspace  VariableName=PV_Generation  SaveFormat=Timeseries  SampleTime=0.01
  To Workspace2 : ToWorkspace  VariableName=SOC  SaveFormat=Timeseries  SampleTime=0.01
  Unit Delay : UnitDelay  SampleTime=-1  HasFrameUpgradeWarning=on
  Unused : Subsystem
  discharging : Constant
  D : Outport
  wires:
  MATLAB Function4/1(P_bess) -> MATLAB Function3/1(P_bess)
  [load_1_P] -> MATLAB Function4/1(P_load), To Workspace/1  "load_consumption"
  [SoC] -> MATLAB Function4/3(SOC), To Workspace2/1
  Constant5/1 -> MATLAB Function4/4(threshold)
  Constant7/1 -> MATLAB Function4/5(max_power)
  Constant8/1 -> MATLAB Function4/7(SOC_max)
  Constant9/1 -> MATLAB Function4/6(SOC_min)
  MATLAB Function3/1(mode) -> Mode/1
  [Vdc_meas_2] -> MATLAB Function6/1(Vdc), MATLAB Function3/3(Vdc), MATLAB Function5/1(Vdc)
  Switch/1 -> Duty cycle/1, Unit Delay/1
  Constant3/1 -> MATLAB Function4/8(efficiency)
  Constant/1 -> Switch1/1
  MATLAB Function4/2(disconnect_flag) -> Switch1/2
  [p_pv] -> To Workspace1/1, MATLAB Function4/2(P_pv)
  discharging/1 -> Manual Switch/1
  Charging/1 -> Manual Switch/2
  From Workspace/1 -> MATLAB Function4/11(dynamic_tariff)
  [V_batt] -> MATLAB Function5/2(Vbatt), MATLAB Function6/2(Vbatt)
  [I_batt] -> MATLAB Function5/3(I_batt_meas), MATLAB Function6/3(I_batt_meas)
  Constant11/1 -> MATLAB Function6/4(I_batt_ref_mag), MATLAB Function5/4(I_batt_ref_mag)
  Constant10/1 -> MATLAB Function6/5(Ts), MATLAB Function5/5(Ts)
  MATLAB Function6/1(D) -> Switch/1
  MATLAB Function5/1(D) -> Switch/3
  Manual Switch/1 -> Switch/2
  Unit Delay/1 -> D/1

== system Microgrid_w_BESS/BESS/Inverter ON//OFF Logic ==
  V_DC : Inport
  g_in : Inport  Port=2
  Compare To Constant : simulink/Logic and Bit Operations/Compare To Constant  relop=>  const=0  OutDataTypeStr=boolean
  Data Type Conversion : DataTypeConversion  OutDataTypeStr=double  SaturateOnIntegerOverflow=off  RndMeth=Floor
  Product : Product
  Unit Delay : UnitDelay  SampleTime=-1  HasFrameUpgradeWarning=on
  g_out : Outport
  wires:
  Data Type Conversion/1 -> Product/1
  V_DC/1 -> Compare To Constant/1
  Compare To Constant/1 -> Data Type Conversion/1
  Product/1 -> Unit Delay/1
  g_in/1 -> Product/2
  Unit Delay/1 -> g_out/1

== system Microgrid_w_BESS/BESS/Subsystem ==
  C_out_1 : spsParallelRLCBranchLib/Parallel RLC Branch  LConnTagsString=a  RConnTagsString=__new0  BranchType=RC  Resistance=10  Inductance=1e-3  SetiL0=off  InitialCurrent=0  Capacitance=100e-6  Setx0=off  InitialVoltage=700  Measurements=None
  Voltage Measurement : spsVoltageMeasurementLib/Voltage Measurement  PhasorSimulation=off  OutputType=Complex  PSBequivalent=0
  + : PMIOPort  Side=Right
  - : PMIOPort  Port=2  Side=Right
  tag scope: Vdc_meas_2=global
  wires:
  Voltage Measurement/1 -> [Vdc_meas_2]
  connections:
  Voltage Measurement/LConn2 -- C_out_1/RConn1 -- -/RConn1
  Voltage Measurement/LConn1 -- C_out_1/LConn1 -- +/RConn1

== system Microgrid_w_BESS/BESS/Subsystem20 ==
  Parallel RLC Branch : spsParallelRLCBranchLib/Parallel RLC Branch  LConnTagsString=a  RConnTagsString=__new0  BranchType=RC  Resistance=10  Inductance=1e-3  SetiL0=off  InitialCurrent=0  Capacitance=2e-6  Setx0=off  InitialVoltage=0  Measurements=None
  Parallel RLC Branch1 : spsParallelRLCBranchLib/Parallel RLC Branch  LConnTagsString=a  RConnTagsString=__new0  BranchType=RC  Resistance=10  Inductance=1e-3  SetiL0=off  InitialCurrent=0  Capacitance=2e-6  Setx0=off  InitialVoltage=0  Measurements=None
  Parallel RLC Branch2 : spsParallelRLCBranchLib/Parallel RLC Branch  LConnTagsString=a  RConnTagsString=__new0  BranchType=RC  Resistance=10  Inductance=1e-3  SetiL0=off  InitialCurrent=0  Capacitance=2e-6  Setx0=off  InitialVoltage=0  Measurements=None
  Three-Phase Series RLC Branch1 : spsThreePhaseSeriesRLCBranchLib/Three-Phase Series RLC Branch  LConnTagsString=A|B|C  RConnTagsString=A|B|C  BranchType=L  Resistance=1  Inductance=3*0.8e-3  Capacitance=1e-6  Measurements=None
  A : PMIOPort  Side=Left
  B : PMIOPort  Port=2  Side=Left
  C : PMIOPort  Port=3  Side=Left
  a : PMIOPort  Port=4  Side=Right
  b : PMIOPort  Port=5  Side=Right
  c : PMIOPort  Port=6  Side=Right
  connections:
  Parallel RLC Branch2/LConn1 -- Parallel RLC Branch1/RConn1 -- c/RConn1 -- Three-Phase Series RLC Branch1/RConn3
  Three-Phase Series RLC Branch1/LConn3 -- C/RConn1
  Three-Phase Series RLC Branch1/LConn2 -- B/RConn1
  Three-Phase Series RLC Branch1/LConn1 -- A/RConn1
  Three-Phase Series RLC Branch1/RConn1 -- a/RConn1 -- Parallel RLC Branch2/RConn1 -- Parallel RLC Branch/LConn1
  Three-Phase Series RLC Branch1/RConn2 -- b/RConn1 -- Parallel RLC Branch1/LConn1 -- Parallel RLC Branch/RConn1

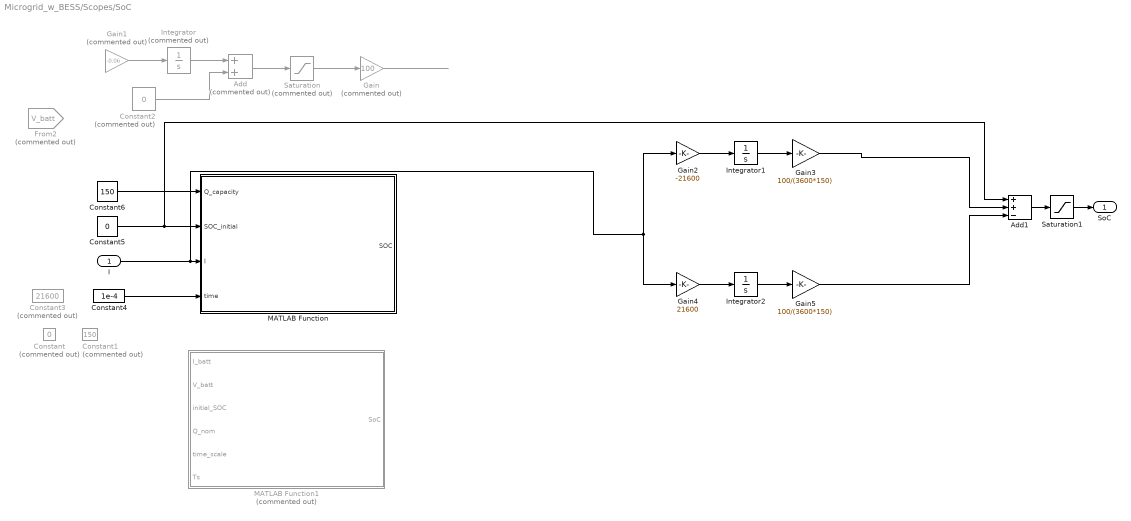
== system Microgrid_w_BESS/Scopes/SoC ==
  I : Inport
  Add : Sum  Commented=on
  Add1 : Sum  Inputs=++-
  Constant : Constant  Commented=on  Value=0
  Constant1 : Constant  Commented=on  Value=150
  Constant2 : Constant  Commented=on  Value=0
  Constant3 : Constant  Commented=on  Value=21600
  Constant4 : Constant  Value=1e-4
  Constant5 : Constant  Value=0
  Constant6 : Constant  Value=150
  From2 : From  Commented=on  GotoTag=V_batt  TagVisibility=global
  Gain : Gain  Commented=on  Gain=100
  Gain1 : Gain  Commented=on  Gain=-0.06
  Gain2 : Gain  Gain=-21600
  Gain3 : Gain  Gain=100/(3600*150)
  Gain4 : Gain  Gain=21600
  Gain5 : Gain  Gain=100/(3600*150)
  Integrator : Integrator  Commented=on
  Integrator1 : Integrator
  Integrator2 : Integrator
  MATLAB Function : MATLAB Function  TreatAsAtomicUnit=on
  MATLAB Function1 : MATLAB Function  Commented=on  TreatAsAtomicUnit=on
  Saturation : Saturate  Commented=on  UpperLimit=1  LowerLimit=0
  Saturation1 : Saturate  UpperLimit=100  LowerLimit=0
  SoC : Outport
  wires:
  Gain1/1 -> Integrator/1
  Add/1 -> Saturation/1
  Integrator/1 -> Add/1
  Saturation/1 -> Gain/1
  Constant2/1 -> Add/2
  Gain/1 -> ?
  Constant4/1 -> MATLAB Function/4(time)
  Constant6/1 -> MATLAB Function/1(Q_capacity)
  Integrator2/1 -> Gain5/1
  Gain3/1 -> Add1/2
  Gain2/1 -> Integrator1/1
  Gain4/1 -> Integrator2/1
  I/1 -> Gain2/1, Gain4/1, MATLAB Function/3(I)
  Gain5/1 -> Add1/3
  Add1/1 -> Saturation1/1
  Integrator1/1 -> Gain3/1
  Constant5/1 -> Add1/1, MATLAB Function/2(SOC_initial)
  Saturation1/1 -> SoC/1

== system Microgrid_w_BESS/Subsystem/Inverter ON//OFF Logic ==
  V_DC : Inport
  g_in : Inport  Port=2
  Compare To Constant : simulink/Logic and Bit Operations/Compare To Constant  relop=>  const=600  OutDataTypeStr=boolean
  Data Type Conversion : DataTypeConversion  OutDataTypeStr=double  SaturateOnIntegerOverflow=off  RndMeth=Floor
  Product : Product
  Unit Delay : UnitDelay  SampleTime=-1  HasFrameUpgradeWarning=on
  g_out : Outport
  wires:
  Data Type Conversion/1 -> Product/1
  V_DC/1 -> Compare To Constant/1
  Compare To Constant/1 -> Data Type Conversion/1
  Product/1 -> Unit Delay/1
  g_in/1 -> Product/2
  Unit Delay/1 -> g_out/1

== system Microgrid_w_BESS/Subsystem/MPPT1 ==
  MATLAB Function1 : MATLAB Function  TreatAsAtomicUnit=on
  PID Controller1 : slpidlib/PID Controller  Controller=PI  Form=Parallel  TimeDomain=Continuous-time  UseExternalTs=off  SampleTime=-1  IntegratorMethod=Forward Euler  FilterMethod=Forward Euler  ControllerParametersSource=internal  P=0.5  I=15*0.002  UseKiTs=on  D=0  UseExternalDerivativeSource=off  N=100  UseFilter=on  TunerSelectOption=Transfer Function Based (PID Tuner App)  InitialConditionSource=internal  InitialConditionForIntegrator=0  InitialConditionForFilter=0  DifferentiatorICPrevScaledInput=0  ExternalReset=none  TrackingMode=off  Kt=1  LimitOutput=off  SatLimitsSource=internal  UpperSaturationLimit=inf  LowerSaturationLimit=-inf  LinearizeAsGain=on  AntiWindupMode=none  Kb=1  LimitIntegrator=off  UpperIntegratorSaturationLimit=inf  LowerIntegratorSaturationLimit=-inf  POutMin=[]  POutMax=[]  IOutMin=[]  IOutMax=[]  DOutMin=[]  DOutMax=[]  NOutMin=[]  NOutMax=[]  SumOutMin=[]  SumOutMax=[]  SaturationOutMin=[]  SaturationOutMax=[]  PParamMin=[]  PParamMax=[]  IParamMin=[]  IParamMax=[]  DParamMin=[]  DParamMax=[]  NParamMin=[]  NParamMax=[]  KbParamMin=[]  KbParamMax=[]  KtParamMin=[]  KtParamMax=[]  KbOutMin=[]  KbOutMax=[]  KtOutMin=[]  KtOutMax=[]  IntegratorOutMin=[]  IntegratorOutMax=[]  FilterOutMin=[]  FilterOutMax=[]  SumI1OutMin=[]  SumI1OutMax=[]  SumI2OutMin=[]  SumI2OutMax=[]  SumI3OutMin=[]  SumI3OutMax=[]  SumI4OutMin=[]  SumI4OutMax=[]  SumDOutMin=[]  SumDOutMax=[]  DifferentiatorOutMin=[]  DifferentiatorOutMax=[]  FilterDiffOutCoefMin=[]  FilterDiffOutCoefMax=[]  ReciprocalOutMin=[]  ReciprocalOutMax=[]  SumDenOutMin=[]  SumDenOutMax=[]  SumNumOutMin=[]  SumNumOutMax=[]  DivideOutMin=[]  DivideOutMax=[]  UdiffTsProdOutMin=[]  UdiffTsProdOutMax=[]  NTsProdOutMin=[]  NTsProdOutMax=[]  UintegralTsProdOutMin=[]  UintegralTsProdOutMax=[]  UngainTsProdOutMin=[]  UngainTsProdOutMax=[]  ClampingZeroOutDataTypeStr=Inherit: Inherit via back propagation  ClampingZeroOutMin=[]  ClampingZeroOutMax=[]  FilterDenConstantOutDataTypeStr=Inherit: Inherit via back propagation  FilterDenConstantOutMin=[]  FilterDenConstantOutMax=[]  PCopyOutDataTypeStr=Inherit: Inherit via back propagation  PCopyOutMin=[]  PCopyOutMax=[]  NCopyOutDataTypeStr=Inherit: Inherit via back propagation  NCopyOutMin=[]  NCopyOutMax=[]  IntegratorContinuousStateAttributes=''  IntegratorStateMustResolveToSignalObject=off  IntegratorRTWStateStorageClass=Auto  FilterContinuousStateAttributes=''  FilterStateMustResolveToSignalObject=off  FilterRTWStateStorageClass=Auto  ParallelPVariant=InternalParameters  IdealPVariant=Disabled  IVariant=InternalParameters  DVariant=Disabled  IntegratorVariant=Continuous  SatVariant=Disabled  AWVariant=Passthrough  PCopyVariant=Disabled  TRVariant=Disabled  FdbkBlocksVariant=Forward  IdealPFdbkVariant=Disabled  SatFdbkVariant=Disabled  DerivativeFilterVariant=Disabled  NVariant=Disabled  NCopyVariant=Disabled_SignalSpec  FilterICVariant=Disabled  IntegratorICVariant=InternalICs  ExternalResetVariant=Disabled  TRSumVariant=Passthrough  SumFdbkVariant=Disabled  SumVariant=Sum_PI  TsampFilterVariant=InternalTs  TsampNgainVariant=Passthrough  TsampIntegralVariant=Disabled_SignalSpec  ExternalSaturationOutDataTypeStr=Inherit: Same as second input  DerivativeSourceVariant=Disabled  PreIntVariant=InternalPreInt
  Saturation : Saturate  UpperLimit=0.392  LowerLimit=0.289
  Sum : Sum  Inputs=|+-
  Unit Delay : UnitDelay  SampleTime=-1  HasFrameUpgradeWarning=on
  D : Outport
  wires:
  PID Controller1/1 -> Saturation/1
  [v_pv_1] -> Sum/2, MATLAB Function1/2(vpv)
  MATLAB Function1/1(Vmpp) -> Sum/1
  [i_pv_1] -> MATLAB Function1/1(ipv)
  Saturation/1 -> Unit Delay/1
  Sum/1 -> PID Controller1/1
  Unit Delay/1 -> D/1

== system Microgrid_w_BESS/Subsystem/Subsystem ==
  C_out_1 : spsParallelRLCBranchLib/Parallel RLC Branch  LConnTagsString=a  RConnTagsString=__new0  BranchType=C  Resistance=10  Inductance=1e-3  SetiL0=off  InitialCurrent=0  Capacitance=1912e-6  Setx0=off  InitialVoltage=700  Measurements=None
  Voltage Measurement : spsVoltageMeasurementLib/Voltage Measurement  PhasorSimulation=off  OutputType=Complex  PSBequivalent=0
  + : PMIOPort  Side=Right
  - : PMIOPort  Port=2  Side=Right
  tag scope: Vdc_meas_1=global
  wires:
  Voltage Measurement/1 -> [Vdc_meas_1]
  connections:
  Voltage Measurement/LConn2 -- C_out_1/RConn1 -- -/RConn1
  Voltage Measurement/LConn1 -- C_out_1/LConn1 -- +/RConn1

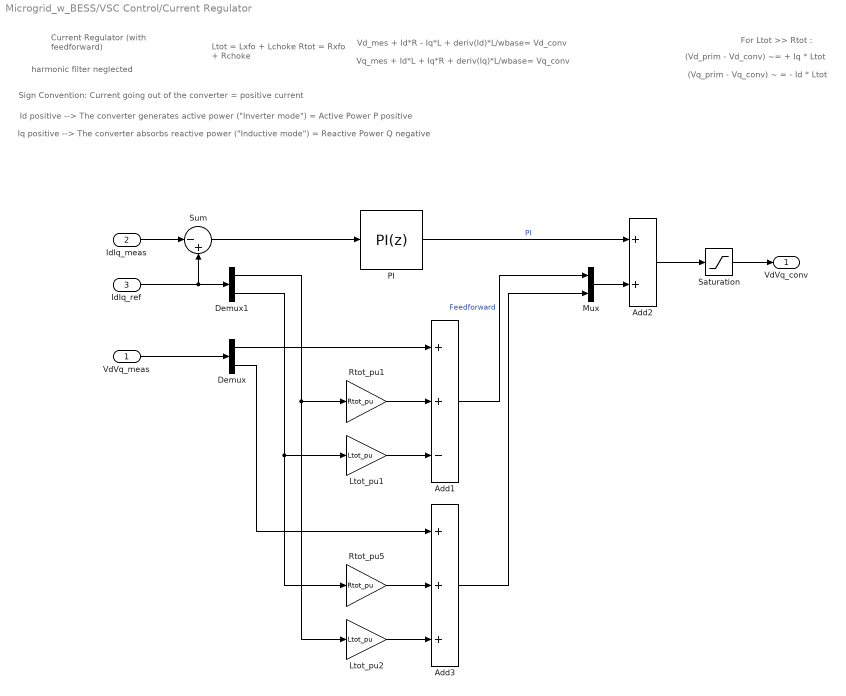
== system Microgrid_w_BESS/VSC Control/Current Regulator ==
  note: For Ltot >> Rtot :
  note: (Vq_prim - Vq_conv) ~ = - Id * Ltot
  note: (Vd_prim - Vd_conv) ~= + Iq * Ltot
  note: Ltot = Lxfo + Lchoke
      | Rtot = Rxfo + Rchoke
  note: Id positive --> The converter generates active power ("Inverter mode") = Active Power P positive
  note: Iq positive --> The converter absorbs reactive power ("Inductive mode") = Reactive Power Q negative
  note: Sign Convention: Current going out of the converter = positive current
  note: Current Regulator
      | (with feedforward)
  note: Vq_mes + Id*L + Iq*R + deriv(Iq)*L/wbase= Vq_conv
  note: Vd_mes + Id*R - Iq*L + deriv(Id)*L/wbase= Vd_conv
  note: harmonic filter neglected
  VdVq_meas : Inport  PortDimensions=2
  IdIq_meas : Inport  Port=2  PortDimensions=2
  IdIq_ref : Inport  Port=3  PortDimensions=2
  Add1 : Sum  Inputs=++-
  Add2 : Sum
  Add3 : Sum  Inputs=+++
  Demux : Demux  Outputs=2
  Demux1 : Demux  Outputs=2
  Ltot_pu1 : Gain  Gain=Ltot_pu  SaturateOnIntegerOverflow=on  OutDataTypeStr=Inherit: Same as input  ParamDataTypeStr=Inherit: Same as input
  Ltot_pu2 : Gain  Gain=Ltot_pu  SaturateOnIntegerOverflow=on  OutDataTypeStr=Inherit: Same as input  ParamDataTypeStr=Inherit: Same as input
  Mux : Mux  Inputs=2
  PI : slpidlib/PID Controller  Controller=PI  Form=Parallel  TimeDomain=Discrete-time  UseExternalTs=off  SampleTime=Ts  IntegratorMethod=Forward Euler  FilterMethod=Forward Euler  ControllerParametersSource=internal  P=Kp_Ireg  I=Ki_Ireg  UseKiTs=off  D=0  UseExternalDerivativeSource=off  N=100  UseFilter=on  TunerSelectOption=Transfer Function Based (PID Tuner App)  InitialConditionSource=internal  InitialConditionForIntegrator=0  InitialConditionForFilter=0  DifferentiatorICPrevScaledInput=0  ExternalReset=none  TrackingMode=off  Kt=1  LimitOutput=on  SatLimitsSource=internal  UpperSaturationLimit=2  LowerSaturationLimit=-2  LinearizeAsGain=off  AntiWindupMode=none  Kb=1  LimitIntegrator=off  UpperIntegratorSaturationLimit=inf  LowerIntegratorSaturationLimit=-inf  POutMin=[]  POutMax=[]  IOutMin=[]  IOutMax=[]  DOutMin=[]  DOutMax=[]  NOutMin=[]  NOutMax=[]  SumOutMin=[]  SumOutMax=[]  SaturationOutMin=[]  SaturationOutMax=[]  PParamMin=[]  PParamMax=[]  IParamMin=[]  IParamMax=[]  DParamMin=[]  DParamMax=[]  NParamMin=[]  NParamMax=[]  KbParamMin=[]  KbParamMax=[]  KtParamMin=[]  KtParamMax=[]  KbOutMin=[]  KbOutMax=[]  KtOutMin=[]  KtOutMax=[]  IntegratorOutMin=[]  IntegratorOutMax=[]  FilterOutMin=[]  FilterOutMax=[]  SumI1OutMin=[]  SumI1OutMax=[]  SumI2OutMin=[]  SumI2OutMax=[]  SumI3OutMin=[]  SumI3OutMax=[]  SumI4OutMin=[]  SumI4OutMax=[]  SumDOutMin=[]  SumDOutMax=[]  DifferentiatorOutMin=[]  DifferentiatorOutMax=[]  FilterDiffOutCoefMin=[]  FilterDiffOutCoefMax=[]  ReciprocalOutMin=[]  ReciprocalOutMax=[]  SumDenOutMin=[]  SumDenOutMax=[]  SumNumOutMin=[]  SumNumOutMax=[]  DivideOutMin=[]  DivideOutMax=[]  UdiffTsProdOutMin=[]  UdiffTsProdOutMax=[]  NTsProdOutMin=[]  NTsProdOutMax=[]  UintegralTsProdOutMin=[]  UintegralTsProdOutMax=[]  UngainTsProdOutMin=[]  UngainTsProdOutMax=[]  ClampingZeroOutDataTypeStr=Inherit: Inherit via back propagation  ClampingZeroOutMin=[]  ClampingZeroOutMax=[]  FilterDenConstantOutDataTypeStr=Inherit: Inherit via back propagation  FilterDenConstantOutMin=[]  FilterDenConstantOutMax=[]  PCopyOutDataTypeStr=Inherit: Inherit via back propagation  PCopyOutMin=[]  PCopyOutMax=[]  NCopyOutDataTypeStr=Inherit: Inherit via back propagation  NCopyOutMin=[]  NCopyOutMax=[]  IntegratorContinuousStateAttributes=''  IntegratorStateMustResolveToSignalObject=off  IntegratorRTWStateStorageClass=Auto  FilterContinuousStateAttributes=''  FilterStateMustResolveToSignalObject=off  FilterRTWStateStorageClass=Auto  ParallelPVariant=InternalParameters  IdealPVariant=Disabled  IVariant=InternalParameters  DVariant=Disabled  IntegratorVariant=Discrete  SatVariant=Enabled  AWVariant=Passthrough  PCopyVariant=Disabled  TRVariant=Disabled  FdbkBlocksVariant=Forward  IdealPFdbkVariant=Disabled  SatFdbkVariant=Disabled  DerivativeFilterVariant=Disabled  NVariant=Disabled  NCopyVariant=Disabled_SignalSpec  FilterICVariant=Disabled  IntegratorICVariant=InternalICs  ExternalResetVariant=Disabled  TRSumVariant=Passthrough  SumFdbkVariant=Disabled  SumVariant=Sum_PI  TsampFilterVariant=InternalTs  TsampNgainVariant=Passthrough  TsampIntegralVariant=Disabled_SignalSpec  ExternalSaturationOutDataTypeStr=Inherit: Same as second input  DerivativeSourceVariant=Disabled  PreIntVariant=InternalPreInt
  Rtot_pu1 : Gain  Gain=Rtot_pu  SaturateOnIntegerOverflow=on  OutDataTypeStr=Inherit: Same as input  ParamDataTypeStr=Inherit: Same as input
  Rtot_pu5 : Gain  Gain=Rtot_pu  SaturateOnIntegerOverflow=on  OutDataTypeStr=Inherit: Same as input  ParamDataTypeStr=Inherit: Same as input
  Saturation : Saturate  UpperLimit=2  LowerLimit=-2
  Sum : Sum  Inputs=|-+
  VdVq_conv : Outport  VectorParamsAs1DForOutWhenUnconnected=off
  wires:
  Add3/1 -> Mux/2
  Demux/2 -> Add3/1
  Add1/1 -> Mux/1  "Feedforward"
  Ltot_pu2/1 -> Add3/3
  Rtot_pu5/1 -> Add3/2
  Demux1/2 -> Rtot_pu5/1, Ltot_pu1/1
  Ltot_pu1/1 -> Add1/3
  Demux1/1 -> Ltot_pu2/1, Rtot_pu1/1
  Rtot_pu1/1 -> Add1/2
  Demux/1 -> Add1/1
  VdVq_meas/1 -> Demux/1
  Saturation/1 -> VdVq_conv/1
  Add2/1 -> Saturation/1
  IdIq_meas/1 -> Sum/1
  IdIq_ref/1 -> Demux1/1, Sum/2
  Sum/1 -> PI/1
  PI/1 -> Add2/1  "PI"
  Mux/1 -> Add2/2

== system Microgrid_w_BESS/VSC Control/Inverter ON//OFF Logic ==
  V_DC : Inport
  AND : Logic  Operator=NAND  IconShape=distinctive  AllPortsSameDT=off  OutDataTypeStr=boolean
  Compare To Constant : simulink/Logic and Bit Operations/Compare To Constant  relop=>=  const=200  OutDataTypeStr=boolean
  Constant : Constant
  Data Type Conversion : DataTypeConversion  OutDataTypeStr=double  SaturateOnIntegerOverflow=off  RndMeth=Floor
  BL : Outport
  tag scope: inv_cont_1=global
  wires:
  Data Type Conversion/1 -> [inv_cont_1], BL/1
  V_DC/1 -> Compare To Constant/1
  AND/1 -> Data Type Conversion/1
  Compare To Constant/1 -> AND/1
  Constant/1 -> AND/2

== system Microgrid_w_BESS/VSC Control/PLL & Measurements ==
  Vabc_prim : Inport
  Iabc_prim : Inport  Port=2
  PLL : powerlib_extras/Discrete  Control Blocks/Discrete 3-phase PLL  Fmin=45  Par_Init="[-0.57  Fnom]"  ParK=[60 1400]  Ts=Ts  AGC=off
  Selector1 : Selector  InputPortWidth=3  IndexOptions=Index vector (dialog)  Indices=[1 2]  OutputSizes=1
  Selector2 : Selector  InputPortWidth=3  IndexOptions=Index vector (dialog)  Indices=[1 2]  OutputSizes=1
  Terminator : Terminator
  V->pu : Gain  Gain=1/(Vnom_prim*sqrt(2)/sqrt(3))  SaturateOnIntegerOverflow=on  OutDataTypeStr=Inherit: Same as input  ParamDataTypeStr=Inherit: Same as input
  V->pu1 : Gain  Gain=Vnom_prim*sqrt(3)/Pnom/sqrt(2)  SaturateOnIntegerOverflow=on  OutDataTypeStr=Inherit: Same as input  ParamDataTypeStr=Inherit: Same as input
  abc_to_dq0 Transformation1 : powerlib_extras/Measurements/abc_to_dq0 Transformation
  abc_to_dq0 Transformation2 : powerlib_extras/Measurements/abc_to_dq0 Transformation
  wt : Outport  VectorParamsAs1DForOutWhenUnconnected=off
  VdVq_prim : Outport  Port=2  VectorParamsAs1DForOutWhenUnconnected=off
  IdIq_prim : Outport  Port=3  VectorParamsAs1DForOutWhenUnconnected=off
  tag scope: IdIq_prim_1_2=global
  wires:
  PLL/1 -> Terminator/1
  PLL/3 -> abc_to_dq0 Transformation1/2, abc_to_dq0 Transformation2/2
  Selector1/1 -> IdIq_prim/1, [IdIq_prim_1_2]
  Selector2/1 -> VdVq_prim/1
  abc_to_dq0 Transformation1/1 -> Selector2/1
  Iabc_prim/1 -> V->pu1/1
  Vabc_prim/1 -> V->pu/1
  PLL/2 -> wt/1
  abc_to_dq0 Transformation2/1 -> Selector1/1
  V->pu/1 -> abc_to_dq0 Transformation1/1, PLL/1
  V->pu1/1 -> abc_to_dq0 Transformation2/1
